simulink model "stepperMotorControl_driver"  (R2021b)
settings: Solver=VariableStepAuto  StartTime=0.0  StopTime=0.1  MaxStep=Ts  RelTol=1e-3
InitFcn:
  | f_pwm = 40e3;
  | Ts = 1e-7;
  | 
  | Reference = 13;
  | t_des = 0.1;
  | 
  | Loaded = 0;
undefined symbols (not defined in the file): Down, Up
libraries: nesl_utility x20, fl_lib x18, ee_lib x5, eePwmGenerator x2
settings Model: Creator=andre  LastModifiedBy=andre

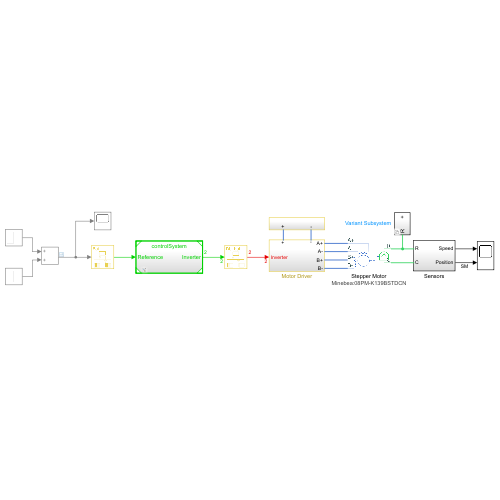
[thumbnail: Simulink's stored preview of the top-level diagram]
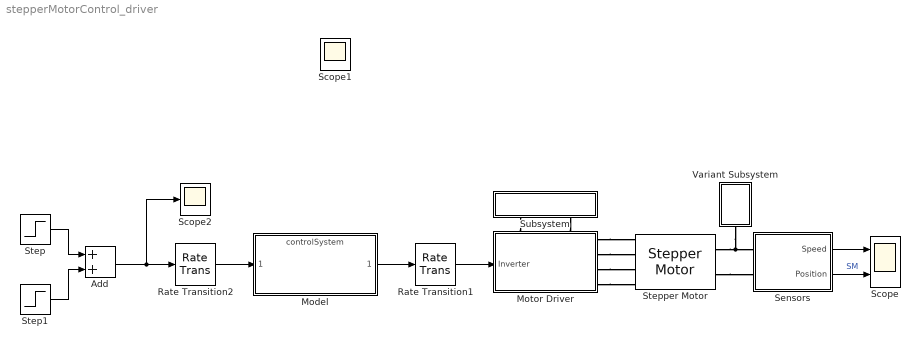
== system stepperMotorControl_driver ==
  Add : Sum
  Model : ModelReference  ModelNameDialog=controlSystem.slx  SimulationMode=Normal  ModelReferenceVersion=1.14
  Motor Driver : Subsystem
      settings: PortSchema="{\"entries\":[{\"content\":{\"sides\":[{\"content\":{\"connectorIds\":[\"In1\"]},\"type\":\"ConnectorPlacement.EquallySpacedRectSide\",\"uuid\":\"c8af76ca-b365-4822-9f74-5abba56d7552\"},{\"content\":{\"connectorIds\":[\"RConn1\",\"RConn2\",\"RConn3\",\"RConn4\"],\"side\":\"RIGHT\"},\"type\":\"ConnectorPlacement.EquallySpacedRectSide\",\"uuid\":\"5d46f4fc-7194-499a-b012-d22610ae7b03\"},{\"content\":{\"connectorIds\":[\"LConn1\",\"LConn2\"],\"side\":\"TOP\"},\"type\":\"ConnectorPlacement.EquallySpacedRectSide\",\"uuid\":\"e224b5e5-21c2-4b26-b67d-ee670febff56\"}]},\"type\":\"ConnectorPlacement.EquallySpacedConnector\",\"uuid\":\"e61f196c-0893-4318-8bcb-0cdd79af0914\"}],\"packageUris\":[\"http://schema.mathworks.com/mf0/Connector/R2020b\"],\"version\":\"1.0\"}"
  Rate Transition1 : RateTransition  Deterministic=off
  Rate Transition2 : RateTransition  Deterministic=off  OutPortSampleTime=5e-5
  Scope : Scope  NumInputPorts=2
  Scope2 : Scope
  Sensors : Subsystem
  Step : Step  Time=0.02  After=Reference  SampleTime=0
  Step1 : Step  Time=0.4  After=-2*Reference  SampleTime=0
  Stepper Motor : ee_lib/Electromechanical/Reluctance & Stepper/Stepper Motor  Tag={'toolbox/physmod/elec/library/m/ee_lib_parts';'Electromechanical/Reluctance_and_Stepper/Stepper_Motor/Minebea/x08PM_K139BSTDCN.xml'}  step_or_av=ee.enum.electromech.simulationMode.stepping  Ra=6.5 Ohm  La=3.2 mH  Km=51.63 mN*m/A  Td=2.5 mN*m  Rm=Inf Ohm  w_vec=[0 1000 3000] rpm  T_vec=[2 2 1] N*m  assert_if_slipping=ee.enum.assertAction.none  J_total=0.0001 kg*m^2  max_step_rate=10 Hz  Step=1.8 deg  J=2.9e-07 kg*m^2  B=2.65e-05 N*m/(rad/s)  speed0=0 rpm  theta0=0 deg  alpha=[0.00393 0.00393] 1/K  Tmeas=25 degC  Tmeas2=125 degC  T_vec2=[1.7 1.7 0.85] N*m  half_stepping=0  thermal_masses=[100 100] J/K  initial_temperatures=[25 25] degC  rotor_thermal_mass=50 J/K  rotor_initial_temperature=25 degC  Rm_percent_rotor=90
      settings: AttributesFormatString=Minebea:08PM-K139BSTDCN  SourceProductBaseCode=PS  InternalSimscapePortConfiguration="{\"Bottom\":[],\"Left\":[{\"id\":\"pA\",\"label\":\"A+\",\"type\":\"foundation.electrical.electrical\"},{\"id\":\"nA\",\"label\":\"A-\",\"type\":\"foundation.electrical.electrical\"},{\"id\":\"pB\",\"label\":\"B+\",\"type\":\"foundation.electrical.electrical\"},{\"id\":\"nB\",\"label\":\"B-\",\"type\":\"foundation.electrical.electrical\"}],\"Right\":[{\"id\":\"R\",\"label\":\"R\",\"type\":\"foundation.mechanical.rotational.rotational\"},{\"id\":\"C\",\"label\":\"C\",\"type\":\"foundation.mechanical.rotational.rotational\"}],\"Top\":[]}"
  Subsystem : Subsystem
      settings: PortSchema="{\"entries\":[{\"content\":{\"sides\":[{\"content\":{\"connectorIds\":[]},\"type\":\"ConnectorPlacement.EquallySpacedRectSide\",\"uuid\":\"759b6f70-d5c2-42e3-87a7-836850e95b0d\"},{\"content\":{\"connectorIds\":[],\"side\":\"RIGHT\"},\"type\":\"ConnectorPlacement.EquallySpacedRectSide\",\"uuid\":\"2f66b810-a356-4f7d-8e6b-60edb676959c\"},{\"content\":{\"connectorIds\":[],\"side\":\"TOP\"},\"type\":\"ConnectorPlacement.EquallySpacedRectSide\",\"uuid\":\"451600ed-c6c2-4080-aaa0-9eca75d0bb88\"},{\"content\":{\"connectorIds\":[\"RConn1\",\"RConn2\"],\"side\":\"BOTTOM\"},\"type\":\"ConnectorPlacement.EquallySpacedRectSide\",\"uuid\":\"2cb6c416-f6d8-4c64-85df-553038b6af98\"}]},\"type\":\"ConnectorPlacement.EquallySpacedConnector\",\"uuid\":\"b5cbc953-e6d2-44b0-89b1-425b511a6c6a\"}],\"packageUris\":[\"http://schema.mathworks.com/mf0/Connector/R2020b\"],\"version\":\"1.0\"}"
  Variant Subsystem : Subsystem  Variant=on
  Scope1 : Scope
  wires:
  Sensors/2(Position) -> Scope/2  "SM"
  Sensors/1(Speed) -> Scope/1
  Step1/1 -> Add/2
  Step/1 -> Add/1
  Add/1 -> Scope2/1, Rate Transition2/1
  Model/1 -> Rate Transition1/1
  Rate Transition2/1 -> Model/1
  Rate Transition1/1 -> Motor Driver/1(Inverter)
  connections:
  Stepper Motor/RConn1 -- Variant Subsystem/LConn1 -- Sensors/LConn1
  Stepper Motor/RConn2 -- Sensors/LConn2
  Motor Driver/RConn1 -- Stepper Motor/LConn1
  Motor Driver/RConn2 -- Stepper Motor/LConn2
  Motor Driver/RConn3 -- Stepper Motor/LConn3
  Motor Driver/RConn4 -- Stepper Motor/LConn4
  Subsystem/RConn1 -- Motor Driver/LConn1
  Subsystem/RConn2 -- Motor Driver/LConn2

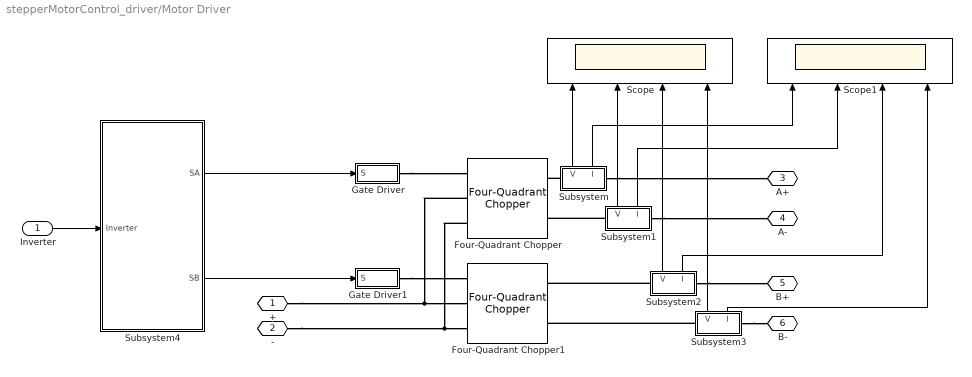
== system stepperMotorControl_driver/Motor Driver ==
  Inverter : Inport
  Four-Quadrant Chopper : ee_lib/Semiconductors & Converters/Converters/Four-Quadrant Chopper  device_type=ee.enum.converters.switchingdevice.mosfet  Vf=0.8 V  Ron=0.001 Ohm  Rds=80e-3 Ohm  Goff=1e-6 1/Ohm  Vth=0.5 V  Vgt=1 V  Vgt_off=-1 V  Ih=1 A  diode_param=ee.enum.converters.protectiondiode.nodynamics  diode_Vf=1 V  diode_Ron=0.001 Ohm  diode_Goff=1e-5 1/Ohm  diode_C=50 nF  diode_iRM=-235 A  diode_iF=300 A  diode_idot=-50 A/us  diode_trr_param=ee.enum.converters.diodetrr.trr_factor  diode_trr_factor=3  diode_trr=15 us  diode_Qrr=1500 s*uA  snubber_type=ee.enum.converters.snubber.exclude  Rs=0.1 Ohm  Cs=1e-7 F
      settings: SourceProductBaseCode=PS  InternalSimscapePortConfiguration="{\"Bottom\":[],\"Left\":[{\"id\":\"G\",\"label\":\"G\",\"type\":\"foundation.electrical.eight_phase\"},{\"id\":\"p1\",\"label\":\"1+\",\"type\":\"foundation.electrical.electrical\"},{\"id\":\"n1\",\"label\":\"1-\",\"type\":\"foundation.electrical.electrical\"}],\"Right\":[{\"id\":\"p2\",\"label\":\"2+\",\"type\":\"foundation.electrical.electrical\"},{\"id\":\"n2\",\"label\":\"2-\",\"type\":\"foundation.electrical.electrical\"}],\"Top\":[]}"
  Four-Quadrant Chopper1 : ee_lib/Semiconductors & Converters/Converters/Four-Quadrant Chopper  device_type=ee.enum.converters.switchingdevice.mosfet  Vf=0.8 V  Ron=0.001 Ohm  Rds=80e-3 Ohm  Goff=1e-6 1/Ohm  Vth=0.5 V  Vgt=1 V  Vgt_off=-1 V  Ih=1 A  diode_param=ee.enum.converters.protectiondiode.nodynamics  diode_Vf=1 V  diode_Ron=0.001 Ohm  diode_Goff=1e-5 1/Ohm  diode_C=50 nF  diode_iRM=-235 A  diode_iF=300 A  diode_idot=-50 A/us  diode_trr_param=ee.enum.converters.diodetrr.trr_factor  diode_trr_factor=3  diode_trr=15 us  diode_Qrr=1500 s*uA  snubber_type=ee.enum.converters.snubber.exclude  Rs=0.1 Ohm  Cs=1e-7 F
      settings: SourceProductBaseCode=PS  InternalSimscapePortConfiguration="{\"Bottom\":[],\"Left\":[{\"id\":\"G\",\"label\":\"G\",\"type\":\"foundation.electrical.eight_phase\"},{\"id\":\"p1\",\"label\":\"1+\",\"type\":\"foundation.electrical.electrical\"},{\"id\":\"n1\",\"label\":\"1-\",\"type\":\"foundation.electrical.electrical\"}],\"Right\":[{\"id\":\"p2\",\"label\":\"2+\",\"type\":\"foundation.electrical.electrical\"},{\"id\":\"n2\",\"label\":\"2-\",\"type\":\"foundation.electrical.electrical\"}],\"Top\":[]}"
  Gate Driver : Subsystem
  Gate Driver1 : Subsystem
  Scope : Scope  NumInputPorts=4
  Scope1 : Scope  NumInputPorts=4
  Subsystem : Subsystem
      settings: PortSchema="{\"entries\":[{\"content\":{\"sides\":[{\"content\":{\"connectorIds\":[\"LConn1\"]},\"type\":\"ConnectorPlacement.EquallySpacedRectSide\",\"uuid\":\"f6ecc8fe-d692-48e4-9862-474903b97fec\"},{\"content\":{\"connectorIds\":[\"RConn1\"],\"side\":\"RIGHT\"},\"type\":\"ConnectorPlacement.EquallySpacedRectSide\",\"uuid\":\"fb2d50ab-b3a3-46bc-9a18-365139e0ba4f\"},{\"content\":{\"connectorIds\":[\"Out1\",\"Out2\"],\"side\":\"TOP\"},\"type\":\"ConnectorPlacement.EquallySpacedRectSide\",\"uuid\":\"c748a75b-7370-4790-bf85-c3d2365a68ca\"}]},\"type\":\"ConnectorPlacement.EquallySpacedConnector\",\"uuid\":\"3f57e7f1-df5d-4a63-9d6a-8189e35da05f\"}],\"packageUris\":[\"http://schema.mathworks.com/mf0/Connector/R2020b\"],\"version\":\"1.0\"}"
  Subsystem1 : Subsystem
      settings: PortSchema="{\"entries\":[{\"content\":{\"sides\":[{\"content\":{\"connectorIds\":[\"LConn1\"]},\"type\":\"ConnectorPlacement.EquallySpacedRectSide\",\"uuid\":\"f6ecc8fe-d692-48e4-9862-474903b97fec\"},{\"content\":{\"connectorIds\":[\"RConn1\"],\"side\":\"RIGHT\"},\"type\":\"ConnectorPlacement.EquallySpacedRectSide\",\"uuid\":\"fb2d50ab-b3a3-46bc-9a18-365139e0ba4f\"},{\"content\":{\"connectorIds\":[\"Out1\",\"Out2\"],\"side\":\"TOP\"},\"type\":\"ConnectorPlacement.EquallySpacedRectSide\",\"uuid\":\"c748a75b-7370-4790-bf85-c3d2365a68ca\"}]},\"type\":\"ConnectorPlacement.EquallySpacedConnector\",\"uuid\":\"3f57e7f1-df5d-4a63-9d6a-8189e35da05f\"}],\"packageUris\":[\"http://schema.mathworks.com/mf0/Connector/R2020b\"],\"version\":\"1.0\"}"
  Subsystem2 : Subsystem
      settings: PortSchema="{\"entries\":[{\"content\":{\"sides\":[{\"content\":{\"connectorIds\":[\"LConn1\"]},\"type\":\"ConnectorPlacement.EquallySpacedRectSide\",\"uuid\":\"f6ecc8fe-d692-48e4-9862-474903b97fec\"},{\"content\":{\"connectorIds\":[\"RConn1\"],\"side\":\"RIGHT\"},\"type\":\"ConnectorPlacement.EquallySpacedRectSide\",\"uuid\":\"fb2d50ab-b3a3-46bc-9a18-365139e0ba4f\"},{\"content\":{\"connectorIds\":[\"Out1\",\"Out2\"],\"side\":\"TOP\"},\"type\":\"ConnectorPlacement.EquallySpacedRectSide\",\"uuid\":\"c748a75b-7370-4790-bf85-c3d2365a68ca\"}]},\"type\":\"ConnectorPlacement.EquallySpacedConnector\",\"uuid\":\"3f57e7f1-df5d-4a63-9d6a-8189e35da05f\"}],\"packageUris\":[\"http://schema.mathworks.com/mf0/Connector/R2020b\"],\"version\":\"1.0\"}"
  Subsystem3 : Subsystem
      settings: PortSchema="{\"entries\":[{\"content\":{\"sides\":[{\"content\":{\"connectorIds\":[\"LConn1\"]},\"type\":\"ConnectorPlacement.EquallySpacedRectSide\",\"uuid\":\"f6ecc8fe-d692-48e4-9862-474903b97fec\"},{\"content\":{\"connectorIds\":[\"RConn1\"],\"side\":\"RIGHT\"},\"type\":\"ConnectorPlacement.EquallySpacedRectSide\",\"uuid\":\"fb2d50ab-b3a3-46bc-9a18-365139e0ba4f\"},{\"content\":{\"connectorIds\":[\"Out1\",\"Out2\"],\"side\":\"TOP\"},\"type\":\"ConnectorPlacement.EquallySpacedRectSide\",\"uuid\":\"c748a75b-7370-4790-bf85-c3d2365a68ca\"}]},\"type\":\"ConnectorPlacement.EquallySpacedConnector\",\"uuid\":\"3f57e7f1-df5d-4a63-9d6a-8189e35da05f\"}],\"packageUris\":[\"http://schema.mathworks.com/mf0/Connector/R2020b\"],\"version\":\"1.0\"}"
  Subsystem4 : Subsystem
  + : PMIOPort  Side=Left
  - : PMIOPort  Port=2  Side=Left
  A+ : PMIOPort  Port=3  Side=Right
  A- : PMIOPort  Port=4  Side=Right
  B+ : PMIOPort  Port=5  Side=Right
  B- : PMIOPort  Port=6  Side=Right
  wires:
  Subsystem/1(V) -> Scope/1
  Subsystem1/1(V) -> Scope/2
  Subsystem2/1(V) -> Scope/3
  Subsystem3/1(V) -> Scope/4
  Subsystem/2(I) -> Scope1/1
  Subsystem1/2(I) -> Scope1/2
  Subsystem2/2(I) -> Scope1/3
  Subsystem3/2(I) -> Scope1/4
  Inverter/1 -> Subsystem4/1(Inverter)
  Subsystem4/1(SA) -> Gate Driver/1(S)
  Subsystem4/2(SB) -> Gate Driver1/1(S)
  connections:
  Gate Driver/RConn1 -- Four-Quadrant Chopper/LConn1
  Gate Driver1/RConn1 -- Four-Quadrant Chopper1/LConn1
  +/RConn1 -- Four-Quadrant Chopper/LConn2 -- Four-Quadrant Chopper1/LConn2
  -/RConn1 -- Four-Quadrant Chopper/LConn3 -- Four-Quadrant Chopper1/LConn3
  Subsystem/LConn1 -- Four-Quadrant Chopper/RConn1
  Subsystem/RConn1 -- A+/RConn1
  Subsystem1/RConn1 -- A-/RConn1
  Subsystem1/LConn1 -- Four-Quadrant Chopper/RConn2
  Subsystem2/RConn1 -- B+/RConn1
  Subsystem2/LConn1 -- Four-Quadrant Chopper1/RConn1
  Subsystem3/RConn1 -- B-/RConn1
  Subsystem3/LConn1 -- Four-Quadrant Chopper1/RConn2

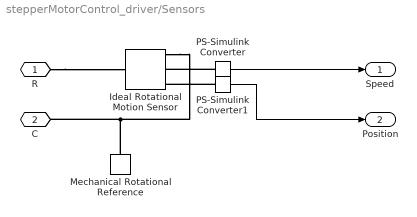
== system stepperMotorControl_driver/Sensors ==
  Ideal Rotational Motion Sensor : fl_lib/Mechanical/Mechanical Sensors/Ideal Rotational Motion Sensor  wrap_angle=simscape.enum.onoff.off  offset=0 rad
  Mechanical Rotational Reference : fl_lib/Mechanical/Rotational Elements/Mechanical Rotational Reference
  PS-Simulink Converter : nesl_utility/PS-Simulink Converter  PhysicalDomain=network_engine_domain  SubClassName=ps_output  LeftPortType=input  RightPortType=output  PseudoPeriodic=off  Frequencies=[]  Unit=rpm  AffineConversion=off
      settings: SourceProductBaseCode=PW,SS
  PS-Simulink Converter1 : nesl_utility/PS-Simulink Converter  PhysicalDomain=network_engine_domain  SubClassName=ps_output  LeftPortType=input  RightPortType=output  PseudoPeriodic=off  Frequencies=[]  Unit=deg  AffineConversion=off
      settings: SourceProductBaseCode=PW,SS
  R : PMIOPort  Side=Left
  C : PMIOPort  Port=2  Side=Left
  Speed : Outport
  Position : Outport  Port=2
  wires:
  PS-Simulink Converter/1 -> Speed/1
  PS-Simulink Converter1/1 -> Position/1
  connections:
  PS-Simulink Converter1/LConn1 -- Ideal Rotational Motion Sensor/RConn3
  Mechanical Rotational Reference/LConn1 -- C/RConn1 -- Ideal Rotational Motion Sensor/RConn1
  PS-Simulink Converter/LConn1 -- Ideal Rotational Motion Sensor/RConn2
  R/RConn1 -- Ideal Rotational Motion Sensor/LConn1

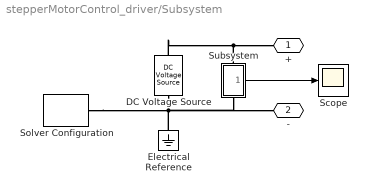
== system stepperMotorControl_driver/Subsystem ==
  DC Voltage Source : fl_lib/Electrical/Electrical Sources/DC Voltage Source  v0=12 V
  Electrical Reference : fl_lib/Electrical/Electrical Elements/Electrical Reference
  Scope : Scope
  Solver Configuration : nesl_utility/Solver Configuration  PhysicalDomain=network_engine_domain  SubClassName=solver  LeftPortType=input  RightPortType=generic  Tones=[]  Harmonics=[]  SimulateNoise=off  Profile=off  UseLocalSampling=off  EnableSwitchedLinearOptims=on  FrequencyDomain=off  UseCCode=off  RelTol=0.001  AbsTol=1e-06  MinStep=1e-09  ToWorkspace=off  RevertToSquareIcSolve=off  NumHomotopyIterations=100  PhasorMode=off  PhasorModeNumHarmonics=1  DoDC=off  ResidualTolerance=1e-09  UseLocalSolver=off  LocalSolverChoice=NE_BACKWARD_EULER_ADVANCER  LocalSolverSampleTime=0.001  DoFixedCost=off  MaxNonlinIter=3  MaxModeIter=2  ComputeImpulses=off  ImpulseIterations=2  LinearAlgebra=auto  EquationFormulation=NE_TIME_EF  DelaysMemoryBudget=1024  AutomaticFiltering=on  FilteringTimeConstant=0.001  PartitionStorageMethod=AS_NEEDED  PartitionMemoryBudget=1024  PartitionMethod=ROBUST
      settings: SourceProductBaseCode=PW,SS
  Subsystem : Subsystem
      settings: PortSchema="{\"entries\":[{\"content\":{\"sides\":[{\"content\":{\"connectorIds\":[\"LConn1\"]},\"type\":\"ConnectorPlacement.EquallySpacedRectSide\",\"uuid\":\"84b439ca-8df1-44b6-8984-f5f279fc989a\"},{\"content\":{\"connectorIds\":[\"RConn1\"],\"side\":\"RIGHT\"},\"type\":\"ConnectorPlacement.EquallySpacedRectSide\",\"uuid\":\"8ccc5838-a74e-4157-a65a-95e55b0daae1\"},{\"content\":{\"connectorIds\":[\"Out1\"],\"side\":\"TOP\"},\"type\":\"ConnectorPlacement.EquallySpacedRectSide\",\"uuid\":\"57e6d481-53f1-4fc4-94d5-e2d87e483097\"}]},\"type\":\"ConnectorPlacement.EquallySpacedConnector\",\"uuid\":\"ae02e184-bf03-425c-8d12-6ab242923918\"}],\"packageUris\":[\"http://schema.mathworks.com/mf0/Connector/R2020b\"],\"version\":\"1.0\"}"
  + : PMIOPort  Side=Right
  - : PMIOPort  Port=2  Side=Right
  wires:
  Subsystem/1(V) -> Scope/1
  connections:
  DC Voltage Source/LConn1 -- Subsystem/LConn1 -- +/RConn1
  DC Voltage Source/RConn1 -- Solver Configuration/RConn1 -- Subsystem/RConn1 -- -/RConn1 -- Electrical Reference/LConn1

== system stepperMotorControl_driver/Variant Subsystem ==
  + : Subsystem  VariantControl=Loaded == 1
  - : Subsystem  VariantControl=Loaded == 0
  R : PMIOPort  Side=Left

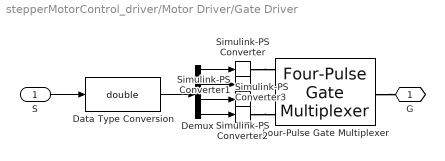
== system stepperMotorControl_driver/Motor Driver/Gate Driver ==
  S : Inport
  Data Type Conversion : DataTypeConversion  OutDataTypeStr=double
  Demux : Demux
  Four-Pulse Gate Multiplexer : ee_lib/Semiconductors & Converters/Converters/Four-Pulse Gate Multiplexer  port_option=ee.enum.controlport.ps
      settings: SourceProductBaseCode=PS  InternalSimscapePortConfiguration="{\"Bottom\":[],\"Left\":[{\"id\":\"G1_ps\",\"label\":\"G1\",\"type\":\"input\"},{\"id\":\"G2_ps\",\"label\":\"G2\",\"type\":\"input\"},{\"id\":\"G3_ps\",\"label\":\"G3\",\"type\":\"input\"},{\"id\":\"G4_ps\",\"label\":\"G4\",\"type\":\"input\"}],\"Right\":[{\"id\":\"p\",\"label\":\"G\",\"type\":\"foundation.electrical.eight_phase\"}],\"Top\":[]}"
  Simulink-PS Converter{,1..3} (4 alike) : nesl_utility/Simulink-PS Converter  PhysicalDomain=network_engine_domain  SubClassName=ps_input  LeftPortType=input  RightPortType=output  PseudoPeriodic=off  Frequencies=[]  NoiseDistribution=none  NoiseParameters=[]  Unit=1  AffineConversion=off  FilteringAndDerivatives=provide  SimscapeFilterOrder=1  InputFilterTimeConstant=0.001  UdotUserProvided=0
      settings: SourceProductBaseCode=PW,SS
  G : PMIOPort  Side=Right
  wires:
  Demux/3 -> Simulink-PS Converter2/1
  Demux/1 -> Simulink-PS Converter/1
  S/1 -> Data Type Conversion/1
  Demux/4 -> Simulink-PS Converter3/1
  Demux/2 -> Simulink-PS Converter1/1
  Data Type Conversion/1 -> Demux/1
  connections:
  Simulink-PS Converter/RConn1 -- Four-Pulse Gate Multiplexer/LConn1
  Simulink-PS Converter2/RConn1 -- Four-Pulse Gate Multiplexer/LConn3
  Simulink-PS Converter3/RConn1 -- Four-Pulse Gate Multiplexer/LConn4
  Simulink-PS Converter1/RConn1 -- Four-Pulse Gate Multiplexer/LConn2
  Four-Pulse Gate Multiplexer/RConn1 -- G/RConn1

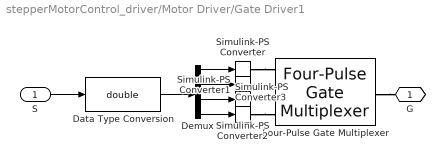
== system stepperMotorControl_driver/Motor Driver/Gate Driver1 ==
  S : Inport
  Data Type Conversion : DataTypeConversion  OutDataTypeStr=double
  Demux : Demux
  Four-Pulse Gate Multiplexer : ee_lib/Semiconductors & Converters/Converters/Four-Pulse Gate Multiplexer  port_option=ee.enum.controlport.ps
      settings: SourceProductBaseCode=PS  InternalSimscapePortConfiguration="{\"Bottom\":[],\"Left\":[{\"id\":\"G1_ps\",\"label\":\"G1\",\"type\":\"input\"},{\"id\":\"G2_ps\",\"label\":\"G2\",\"type\":\"input\"},{\"id\":\"G3_ps\",\"label\":\"G3\",\"type\":\"input\"},{\"id\":\"G4_ps\",\"label\":\"G4\",\"type\":\"input\"}],\"Right\":[{\"id\":\"p\",\"label\":\"G\",\"type\":\"foundation.electrical.eight_phase\"}],\"Top\":[]}"
  Simulink-PS Converter{,1..3} (4 alike) : nesl_utility/Simulink-PS Converter  PhysicalDomain=network_engine_domain  SubClassName=ps_input  LeftPortType=input  RightPortType=output  PseudoPeriodic=off  Frequencies=[]  NoiseDistribution=none  NoiseParameters=[]  Unit=1  AffineConversion=off  FilteringAndDerivatives=provide  SimscapeFilterOrder=1  InputFilterTimeConstant=0.001  UdotUserProvided=0
      settings: SourceProductBaseCode=PW,SS
  G : PMIOPort  Side=Right
  wires:
  Data Type Conversion/1 -> Demux/1
  Demux/2 -> Simulink-PS Converter1/1
  Demux/4 -> Simulink-PS Converter3/1
  S/1 -> Data Type Conversion/1
  Demux/1 -> Simulink-PS Converter/1
  Demux/3 -> Simulink-PS Converter2/1
  connections:
  Four-Pulse Gate Multiplexer/RConn1 -- G/RConn1
  Simulink-PS Converter1/RConn1 -- Four-Pulse Gate Multiplexer/LConn2
  Simulink-PS Converter3/RConn1 -- Four-Pulse Gate Multiplexer/LConn4
  Simulink-PS Converter2/RConn1 -- Four-Pulse Gate Multiplexer/LConn3
  Simulink-PS Converter/RConn1 -- Four-Pulse Gate Multiplexer/LConn1

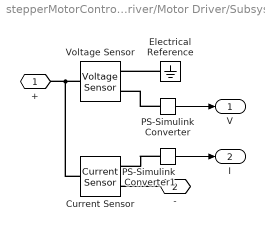
== system stepperMotorControl_driver/Motor Driver/Subsystem ==
  Current Sensor : fl_lib/Electrical/Electrical Sensors/Current Sensor
  Electrical Reference : fl_lib/Electrical/Electrical Elements/Electrical Reference
  PS-Simulink Converter : nesl_utility/PS-Simulink Converter  PhysicalDomain=network_engine_domain  SubClassName=ps_output  LeftPortType=input  RightPortType=output  PseudoPeriodic=off  Frequencies=[]  Unit=V  AffineConversion=off
      settings: SourceProductBaseCode=PW,SS
  PS-Simulink Converter1 : nesl_utility/PS-Simulink Converter  PhysicalDomain=network_engine_domain  SubClassName=ps_output  LeftPortType=input  RightPortType=output  PseudoPeriodic=off  Frequencies=[]  Unit=A  AffineConversion=off
      settings: SourceProductBaseCode=PW,SS
  Voltage Sensor : fl_lib/Electrical/Electrical Sensors/Voltage Sensor
  + : PMIOPort  Side=Left
  - : PMIOPort  Port=2  Side=Right
  V : Outport
  I : Outport  Port=2
  wires:
  PS-Simulink Converter/1 -> V/1
  PS-Simulink Converter1/1 -> I/1
  connections:
  Voltage Sensor/LConn1 -- Current Sensor/LConn1 -- +/RConn1
  PS-Simulink Converter/LConn1 -- Voltage Sensor/RConn1
  Electrical Reference/LConn1 -- Voltage Sensor/RConn2
  -/RConn1 -- Current Sensor/RConn2
  PS-Simulink Converter1/LConn1 -- Current Sensor/RConn1

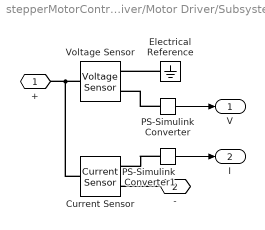
== system stepperMotorControl_driver/Motor Driver/Subsystem1 ==
  Current Sensor : fl_lib/Electrical/Electrical Sensors/Current Sensor
  Electrical Reference : fl_lib/Electrical/Electrical Elements/Electrical Reference
  PS-Simulink Converter : nesl_utility/PS-Simulink Converter  PhysicalDomain=network_engine_domain  SubClassName=ps_output  LeftPortType=input  RightPortType=output  PseudoPeriodic=off  Frequencies=[]  Unit=V  AffineConversion=off
      settings: SourceProductBaseCode=PW,SS
  PS-Simulink Converter1 : nesl_utility/PS-Simulink Converter  PhysicalDomain=network_engine_domain  SubClassName=ps_output  LeftPortType=input  RightPortType=output  PseudoPeriodic=off  Frequencies=[]  Unit=A  AffineConversion=off
      settings: SourceProductBaseCode=PW,SS
  Voltage Sensor : fl_lib/Electrical/Electrical Sensors/Voltage Sensor
  + : PMIOPort  Side=Left
  - : PMIOPort  Port=2  Side=Right
  V : Outport
  I : Outport  Port=2
  wires:
  PS-Simulink Converter1/1 -> I/1
  PS-Simulink Converter/1 -> V/1
  connections:
  PS-Simulink Converter1/LConn1 -- Current Sensor/RConn1
  -/RConn1 -- Current Sensor/RConn2
  Electrical Reference/LConn1 -- Voltage Sensor/RConn2
  PS-Simulink Converter/LConn1 -- Voltage Sensor/RConn1
  Current Sensor/LConn1 -- Voltage Sensor/LConn1 -- +/RConn1

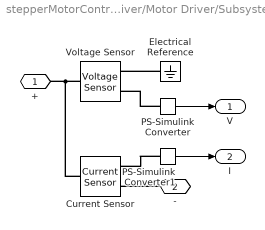
== system stepperMotorControl_driver/Motor Driver/Subsystem2 ==
  Current Sensor : fl_lib/Electrical/Electrical Sensors/Current Sensor
  Electrical Reference : fl_lib/Electrical/Electrical Elements/Electrical Reference
  PS-Simulink Converter : nesl_utility/PS-Simulink Converter  PhysicalDomain=network_engine_domain  SubClassName=ps_output  LeftPortType=input  RightPortType=output  PseudoPeriodic=off  Frequencies=[]  Unit=V  AffineConversion=off
      settings: SourceProductBaseCode=PW,SS
  PS-Simulink Converter1 : nesl_utility/PS-Simulink Converter  PhysicalDomain=network_engine_domain  SubClassName=ps_output  LeftPortType=input  RightPortType=output  PseudoPeriodic=off  Frequencies=[]  Unit=A  AffineConversion=off
      settings: SourceProductBaseCode=PW,SS
  Voltage Sensor : fl_lib/Electrical/Electrical Sensors/Voltage Sensor
  + : PMIOPort  Side=Left
  - : PMIOPort  Port=2  Side=Right
  V : Outport
  I : Outport  Port=2
  wires:
  PS-Simulink Converter/1 -> V/1
  PS-Simulink Converter1/1 -> I/1
  connections:
  +/RConn1 -- Voltage Sensor/LConn1 -- Current Sensor/LConn1
  PS-Simulink Converter/LConn1 -- Voltage Sensor/RConn1
  Electrical Reference/LConn1 -- Voltage Sensor/RConn2
  -/RConn1 -- Current Sensor/RConn2
  PS-Simulink Converter1/LConn1 -- Current Sensor/RConn1

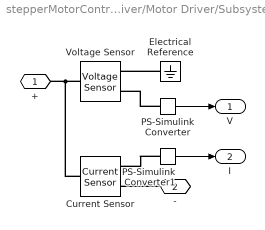
== system stepperMotorControl_driver/Motor Driver/Subsystem3 ==
  Current Sensor : fl_lib/Electrical/Electrical Sensors/Current Sensor
  Electrical Reference : fl_lib/Electrical/Electrical Elements/Electrical Reference
  PS-Simulink Converter : nesl_utility/PS-Simulink Converter  PhysicalDomain=network_engine_domain  SubClassName=ps_output  LeftPortType=input  RightPortType=output  PseudoPeriodic=off  Frequencies=[]  Unit=V  AffineConversion=off
      settings: SourceProductBaseCode=PW,SS
  PS-Simulink Converter1 : nesl_utility/PS-Simulink Converter  PhysicalDomain=network_engine_domain  SubClassName=ps_output  LeftPortType=input  RightPortType=output  PseudoPeriodic=off  Frequencies=[]  Unit=A  AffineConversion=off
      settings: SourceProductBaseCode=PW,SS
  Voltage Sensor : fl_lib/Electrical/Electrical Sensors/Voltage Sensor
  + : PMIOPort  Side=Left
  - : PMIOPort  Port=2  Side=Right
  V : Outport
  I : Outport  Port=2
  wires:
  PS-Simulink Converter1/1 -> I/1
  PS-Simulink Converter/1 -> V/1
  connections:
  PS-Simulink Converter1/LConn1 -- Current Sensor/RConn1
  -/RConn1 -- Current Sensor/RConn2
  Electrical Reference/LConn1 -- Voltage Sensor/RConn2
  PS-Simulink Converter/LConn1 -- Voltage Sensor/RConn1
  Current Sensor/LConn1 -- Voltage Sensor/LConn1 -- +/RConn1

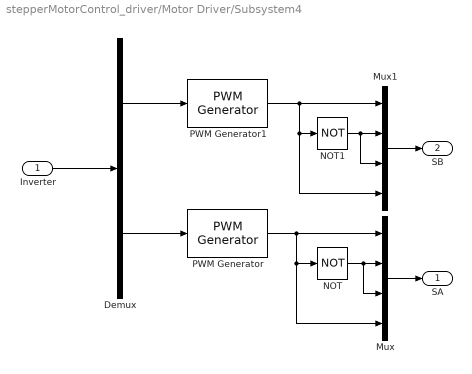
== system stepperMotorControl_driver/Motor Driver/Subsystem4 ==
  Inverter : Inport
  Demux : Demux  Outputs=2
  Mux : Mux
  Mux1 : Mux
  NOT : Logic  Operator=NOT  AllPortsSameDT=off  OutDataTypeStr=boolean
  NOT1 : Logic  Operator=NOT  AllPortsSameDT=off  OutDataTypeStr=boolean
  PWM Generator : eePwmGenerator/PWM Generator  CarrCount=Up-Down  Tper=1/f_pwm  Tdelay=0  Ts=Ts
  PWM Generator1 : eePwmGenerator/PWM Generator  CarrCount=Up-Down  Tper=1/f_pwm  Tdelay=0  Ts=Ts
  SA : Outport
  SB : Outport  Port=2
  wires:
  Mux1/1 -> SB/1
  PWM Generator1/1 -> Mux1/4, NOT1/1, Mux1/1
  Inverter/1 -> Demux/1
  Mux/1 -> SA/1
  NOT/1 -> Mux/3, Mux/2
  PWM Generator/1 -> Mux/1, Mux/4, NOT/1
  NOT1/1 -> Mux1/3, Mux1/2
  Demux/2 -> PWM Generator/1
  Demux/1 -> PWM Generator1/1

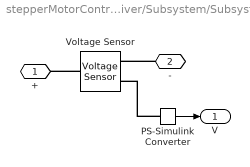
== system stepperMotorControl_driver/Subsystem/Subsystem ==
  PS-Simulink Converter : nesl_utility/PS-Simulink Converter  PhysicalDomain=network_engine_domain  SubClassName=ps_output  LeftPortType=input  RightPortType=output  PseudoPeriodic=off  Frequencies=[]  Unit=V  AffineConversion=off
      settings: SourceProductBaseCode=PW,SS
  Voltage Sensor : fl_lib/Electrical/Electrical Sensors/Voltage Sensor
  + : PMIOPort  Side=Left
  - : PMIOPort  Port=2  Side=Right
  V : Outport
  wires:
  PS-Simulink Converter/1 -> V/1
  connections:
  Voltage Sensor/LConn1 -- +/RConn1
  PS-Simulink Converter/LConn1 -- Voltage Sensor/RConn1
  -/RConn1 -- Voltage Sensor/RConn2

== system stepperMotorControl_driver/Variant Subsystem/+ ==
  Inertia : fl_lib/Mechanical/Rotational Elements/Inertia  inertia=5e-5 kg*m^2  num_ports=foundation.enum.numPorts2.one  w_specify=off  w_priority=High  w=0 rad/s  w_nominal_specify=off  w_nominal_unit=rad/s  w_nominal_value=1  t_specify=off  t_priority=None  t=0 N*m  t_nominal_specify=off  t_nominal_unit=N*m  t_nominal_value=1
  R : PMIOPort  Side=Left
  connections:
  Inertia/LConn1 -- R/RConn1

== system stepperMotorControl_driver/Variant Subsystem/- ==
  R : PMIOPort  Side=Left
